simulink model "BEV_Laengsdynamikmodell_v2"  (R2023b)
settings: configuration reference "SharedConfig" (kept outside this file)
undefined symbols (not defined in the file): acc_cycle_flag, Analyse, battery, battery_builder_rtmsupport, config_battery, config_gearbox, config_Inverter, config_motor, config_vehicle, GB, gcbh, gearbox_map, k_FW, ModuleAssembly1, ModuleType1, motormap, motormap2
libraries: powerlib x37, nesl_utility x18, GD_Batterymodel_NSGAII_1_lib x12, BatteryProtection x9, fl_lib x7, dspstat3 x4, simulink x3, eePmsmCurrentReferenceGen x2, spsControlledCurrentSourceLib x2, spsVoltageMeasurementLib x2, batt_lib x1, BatteryBalancing x1
(part 6 of 6)

== matlab function BEV_Laengsdynamikmodell_v2/Variant Subsystem Inverter/Inverter Analytic/Variant Subsystem/IM_Inverter_SiC-MOSFET_Analytic/C2M0025120D ==
  data: io input; udc input; up input; fs input; CPloss_SiC output; CPloss_diode output; costheta input; SPloss_SiC output; SPloss_diode output; T_mosfet input; T_diode input
function [CPloss_SiC,CPloss_diode,SPloss_SiC,SPloss_diode] = SiC_MOSFET(io,udc,up,fs,costheta,T_mosfet,T_diode)
%%%%%%%%%%%%%%%%%%%%%%%%%%% parameter table %%%%%%%%%%%%%%%%%%%%%%%%%%%%%%%
%%%%%%%%%%%%%%%%%%%%%%%%%%% varialbe table %%%%%%%%%%%%%%%%%%%%%%%%%%%%%%%%
%variavle name      meaning,                                                        unit
%io,                operation current                                               (A)
%up,                operation voltage                                               (V)
%udc,               DC bus voltage,                                                 (V)
%fs,                switching frequency,                                            (Hz)
%costheta,          power factor,                                                   (none)
%CPloss_igbt,       conduction loss on IGBT,                                        (W)
%CPloss_diode,      conduction loss on the reverse paralleled diode,                (W)
%SPloss_igbt,       switching loss on IGBT,                                         (W)
%SPloss_diode,      switching loss on the reverse paralleled diode,                 (W)
%%%%%%%%%%%%%%%%%%%%%%%%%%%%%%%%%%%%%%%%%%%%%%%%%%%%%%%%%%%%%%%%%%%%%%%%%%%
parallel = 4;

io = io/parallel;
rdson_max = 0.02;       
alpha = (1.45 - 1)/(150 - 25);
ud_plateau25 = 1;                              % Fig.11; Vth,25 = 2.7
ud_plateau150 = 0.717;                         % Fig.11; Vth,150 = 2.3
%%%%%%%%%%%%%%%%%%%%%%%%%%%% linearization %%%%%%%%%%%%%%%%%%%%%%%%%%%%%%%%
rdson = rdson_max*(1 + alpha/100)^(T_mosfet - 25);
ud_plateau = ud_plateau25 + (ud_plateau25-ud_plateau150)/(25-150)*(T_diode-25);

rd = (-6 - (-3.75))/(-200 - 0) * 1.2;          % engineering calculation use safty margin value, linearization from Fig.10, using Vsd,typ = 3.5;

Eon_SiC = (0.00069/80*(io*(2/pi)))/520*udc;    % linearization from Fig.23; V_DD = 600; Eon(60, 0.0015);
Eoff_SiC = (0.001125/80*(io*(2/pi)))/520*udc;  % linearization from Fig.23; V_DD = 600; Eoff(60, 0.00075);
Eon_diode = 0;
Eoff_diode = 0;
%%%%%%%%%%%%%%%%%%%%%%%%%%%%%%%%%%%%%%%%%%%%%%%%%%%%%%%%%%%%%%%%%%%%%%%%%%%
m = sqrt(2)*up*2/udc;

if io*rdson <= ud_plateau
   CPloss_SiC = rdson*io^2;
   CPloss_diode = 0;
   SPloss_SiC = fs*(Eon_SiC+Eoff_SiC);
   SPloss_diode = fs*(Eon_diode+Eoff_diode);
else
   CPloss_SiC = 2*rdson*io*io*(1/8+m*costheta/3/pi);
   CPloss_diode = sqrt(2)*ud_plateau*io*(1/2/pi-m*costheta/8)+2*rd*io*io*(1/8-m*costheta/3/pi);
   SPloss_SiC = fs*(Eon_SiC+Eoff_SiC);
   SPloss_diode = fs*(Eon_diode+Eoff_diode);
end

CPloss_SiC = CPloss_SiC*parallel;
SPloss_SiC = SPloss_SiC*parallel;
CPloss_diode = CPloss_diode*parallel;
SPloss_diode = SPloss_diode*parallel;

if io == 0
   SPloss_SiC = 0;
   SPloss_diode = 0;
end
end

== matlab function BEV_Laengsdynamikmodell_v2/MATLAB Function1 ==
  data: u input
function fcn(u)
%disp('rpm:')
%disp (u)

== matlab function BEV_Laengsdynamikmodell_v2/Variant Subsystem Gearbox/Gearbox Analytic/Oil Temp/MATLAB Function ==
  data: t input; P_V input; T output
function T = fcn(t, P_V)

coder.extrinsic('evalin');

% Calculate lubricant temperature
ambient_temp = 0;
ambient_temp = evalin('base', 'config_vehicle.ambient_temp');
% 
% if t < (ambient_temp - 273)
%     T = (ambient_temp - 273);
% elseif t <= 70 %Aufwärmphase mit Umgebung < t < 70°C
%     T = abs(P) * 0.0003 + rpm * 0.00004 + t; %Leistungsabhängiger und drehzahlabhängiger Energieeintrag (Temperaturanstieg)
% else %Temperatur t > 70°C -> Wärmeabgabe ~ delta_t und ~ delta_t^2 (mit delta_t = t_gearbox - t_ambient)
%     T = abs(P) * 0.0003 + rpm * 0.00004 + t - (t - ambient_temp + 273) * 0.0002 - (t - ambient_temp + 273)^2 * 0.0000022;
% end

if t < (ambient_temp - 273)
    T = (ambient_temp - 273);
elseif t <= 80 %Aufwärmphase mit Umgebung < t < 70°C
    T =0.000055*P_V + t - (t - ambient_temp + 273) * 0.0003; %Leistungsabhängiger und drehzahlabhängiger Energieeintrag (Temperaturanstieg)
else %Temperatur t > 70°C -> Wärmeabgabe ~ delta_t und ~ delta_t^2 (mit delta_t = t_gearbox - t_ambient)
    T = 0.000088*P_V + t - (t - ambient_temp + 273) * 0.0010 - (t - ambient_temp + 273)^2 * 0.000012;
end

end

== matlab function BEV_Laengsdynamikmodell_v2/Variant Subsystem Inverter/Inverter Analytic/Variant Subsystem/IM_Inverter_SiC-MOSFET_Analytic/MATLAB Function3 ==
  data: u output; T_m input; i output; usq input; usd input; costheta output; n input
function [u, i, costheta] = fcn(T_m, usq, usd, n)

   Lm = 4.5e-4;
   Lr =  0.01571 + Lm;
   p = 3;
   T_e = T_m/p;
   
   if T_m >=0
       id = -sqrt((2*T_e/p*Lr)/(3*p*Lm^2));
   else
       id = sqrt((-2*T_e/p*Lr)/(3*p*Lm^2));
   end
   iq = id;
   i = sqrt(id^2 + iq^2)/2;
   u = sqrt(usq*usq+usd*usd);
   costheta = (usd*id+usq*iq)/u/i;

   if isnan(costheta)
       costheta = 1;
   end

   if n < 0.1
       u = 0;
       i = 0;
       costheta = 1;
   end

end

== matlab function BEV_Laengsdynamikmodell_v2/Current_fix/MATLAB Function3 ==
  data: state input; u input; y output; st output
function [y, st] = fcn(state, u)
z = 0;
st = 0;
u = double(u);

coder.extrinsic('evalin');

z = evalin('base', 'acc_cycle_flag');
if state == 1
    y = state;
else
    if (u == 1) && (z == 1)
        warning("Battery: Voltage went below 0V - Quiting battery simulation for acceleration-cycle")
    elseif (u == 1) && (z ~= 1)
        warning("Battery: Voltage went below 0V - Battery failed in Main Drivingcycle - Stopping simulation")
        st = 1;
    end
    y = u;
end

== matlab function BEV_Laengsdynamikmodell_v2/Variant Subsystem Battery/Battery simplified (R0)/Battery/MATLAB Function3 ==
  settings: updateMethod=DISCRETE
  data: car_current input; parallel_cells input; V0_matCell input; iCell output; numCyclesCell output; socCell output; socParallelAssembly output; temperatureCell output; vCell output; vParallelAssembly output; R0_matCell input; AH_Cell input; thermal_massCell input; AmbientResistance input; InitialSOC input; T_battery input; SOC_vecCell input; T_vecCell input; T_ambient input; time input; P_bat_loss output
function [iCell, numCyclesCell, socCell, socParallelAssembly, temperatureCell, vCell, vParallelAssembly, P_bat_loss] = fcn(car_current, parallel_cells, V0_matCell, R0_matCell, AH_Cell, ...
    thermal_massCell, AmbientResistance, InitialSOC, T_battery, SOC_vecCell, T_vecCell, T_ambient, time)

    % Initialize Parameters
    dt = 1;  % Time step in seconds
    T_target_inital = 298.15;
    alpha = 1.25e-4;
    T_target = T_target_inital + alpha * time;  % Target temperature in K (e.g., 25°C)
    K_p = 0.1;  % Proportional gain for PI controller
    K_i = 0.01;  % Integral gain for PI control
    persistent numCyclesCell_previous soc_previous T_battery_previous integral_error;

    if isempty(soc_previous)
        soc_previous = InitialSOC;  % Set initial state of charge
        numCyclesCell_previous = 0;  % Initial number of cycles
        T_battery_previous = T_battery;  % Initial battery temperature
        integral_error = 0;  % Initialize integral term for PI control
    end

    % Battery Current (car_current as input)
    iCell = car_current / parallel_cells;  % Current flowing through each cell

    % Update State of Charge using Coulomb counting
    if iCell ~= 0
        socCell = soc_previous - (-iCell * dt / (3600 * AH_Cell));  % Updated SOC
    else
        socCell = soc_previous;  % No change if no current
    end
    socCell = max(0, min(socCell, 1));  % Ensure SOC stays within valid range [0, 1]

    % Update cycle count
    delta_soc = soc_previous - socCell;
    numCyclesIncrement = max(0, delta_soc);
    numCyclesCell_previous = numCyclesCell_previous + numCyclesIncrement;
    numCyclesCell = numCyclesCell_previous;
    socParallelAssembly = socCell;

    % Heat Transfer Calculations
    Q_ambient = (T_battery_previous - T_ambient) / AmbientResistance;

    % PI control for dynamic mass flow rate
    error = T_battery_previous - T_target;
    integral_error = integral_error + error * dt;
    mass_dot = max(0, K_p * error + K_i * integral_error);

    % Maximum mass flow rate limit
    Re = 2000; % Laminar flow
    mu = 8.9e-4; % Dynamic viscosity of water
    density = 1000; % Density of water
    D_h = 0.005; % Hydraulic diameter of pipe
    n = 4; % Number of channels
    A = (pi * n * D_h^2) / 4; % Cross-sectional area of channels
    cp = 4184; % Specific heat capacity of water
    v = (Re * mu) / (density * D_h); % Flow velocity of coolant
    
    mass_dot_max = density * A * v;
    mass_dot = min(mass_dot, mass_dot_max);

    Delta_T_initial = 0.03;   % Initial jump in temperature difference
    Delta_T_max = 0.04;       % Maximum temperature difference at steady state
    tau = 10;                 % Time constant, adjust based on system behavior
    beta = 4e-5;
    Temp_difference = Delta_T_initial + (Delta_T_max - Delta_T_initial) * (1 - exp(-time / tau)) + beta*time;

    Q_coolant = mass_dot * cp * Temp_difference;
    Q_total = Q_coolant + Q_ambient;

    % Iterative temperature calculation
    tolerance = 1e-3;
    max_iterations = 100;
    T_battery_new = T_battery_previous;
    iteration = 0;

    while true
        R0_interpolated = interp2(T_vecCell, SOC_vecCell, R0_matCell, T_battery_new, socCell, 'linear');

        % Heat generated
        Q_generated = iCell^2 * (R0_interpolated);
        dT_battery_dt = (Q_generated - Q_total) / thermal_massCell;
        T_battery_new_next = T_battery_previous + dT_battery_dt * dt;

        % Check convergence
        if abs(T_battery_new_next - T_battery_new) < tolerance
            break;
        end
        T_battery_new = T_battery_new_next;
        iteration = iteration + 1;

        if iteration >= max_iterations
            warning('Temperature calculation did not converge within max iterations');
            break;
        end
    end

    T_battery_new = T_battery_new_next;
    temperatureCell = T_battery_new;

    % Interpolated OCV
    V0_interpolated = interp2(T_vecCell, SOC_vecCell, V0_matCell, T_battery_new, socCell, 'linear');

    % Calculate vCell including dynamic effects
    vCell = V0_interpolated - (-iCell * R0_interpolated);

    % Voltage for Parallel Assembly
    vParallelAssembly = vCell;

    % Update previous state variables for the next time step
    soc_previous = socCell;
    T_battery_previous = T_battery_new;
    
    % Ohmic losses
    Q_ohmic = Q_generated;
    % Total losses
    Q_total_loss = Q_ohmic;
    
    P_bat_loss = Q_total_loss;


end

== matlab function BEV_Laengsdynamikmodell_v2/MATLAB Function2 ==
  data: u input
function fcn(u)
%disp('torque')
%disp (u)

== matlab function BEV_Laengsdynamikmodell_v2/Variant Subsystem Inverter/Inverter Simple/MATLAB Function ==
  data: P_inv_loss output; I_dc output; T input; n input; udc input; P_inv_total output; P_mot_total output; P_Terminal input
function [P_inv_loss, I_dc, P_inv_total, P_mot_total]= fcn(T, n, udc, P_Terminal)

    correction_faktor = 1;

    P_inv_total = P_Terminal;
    I_dc = P_inv_total/udc;
    P_mot_total = (2*T*pi*n/60+P_inv_total)/2;
    P_inv_loss = correction_faktor * (P_inv_total - P_mot_total);

end

== matlab function BEV_Laengsdynamikmodell_v2/Variant Subsystem Gearbox/Gearbox Lookup-Table/Oil Temp Gao/MATLAB Function ==
  data: t input; P input; T output; rpm input
function T = fcn(t, P, rpm)

coder.extrinsic('evalin');

% Calculate lubricant temperature
ambient_temp = 0;
ambient_temp = evalin('base', 'config_vehicle.ambient_temp');

% if t < (ambient_temp - 273)
%     T = (ambient_temp - 273);
% elseif t <= 75
%     T = abs(P) * 0.005 + t - (t - ambient_temp + 273)* 0.001;
% else
%     T = abs(P) * 0.005 + t - (t - 75) * 0.002 - (t - ambient_temp + 273)* 0.001;
% end

if t < (ambient_temp - 273)
    T = (ambient_temp - 273);
elseif t <= 70 %Aufwärmphase mit Umgebung < t < 70°C
    T = abs(P) * 0.0003 + rpm * 0.00004 + t; %Leistungsabhängiger und drehzahlabhängiger Energieeintrag (Temperaturanstieg)
else %Temperatur t > 70°C -> Wärmeabgabe ~ delta_t und ~ delta_t^2 (mit delta_t = t_gearbox - t_ambient)
    T = abs(P) * 0.0003 + rpm * 0.00004 + t - (t - ambient_temp + 273) * 0.0002 - (t - ambient_temp + 273)^2 * 0.0000022;
end

end

== matlab function BEV_Laengsdynamikmodell_v2/Variant Subsystem Gearbox/Gearbox Analytic/Variant Subsystem Analytic GB/Zweistufig_Koaxial/MATLAB Function ==
  data: P_V output double size=1; Mrad input; nrad input; Temp input; GB parameter
function P_V = Getriebe_Einstufig_Achsparallel(Mrad, nrad, Temp, GB)

if nrad == 0
    P_V = 0;
else
    P_V = Getrieberechnung_koaxial(GB,Mrad,nrad,Temp);
end

end

== matlab function BEV_Laengsdynamikmodell_v2/Variant Subsystem Motor/Motor Lookup-Table/MATLAB Function2 ==
  data: u input; y output
function y = fcn(u)

if isnan(u)
    warning('P_motor_111 is NaN. Setting it to 0.');
    y = 0;
else
    y = u;
end

== matlab function BEV_Laengsdynamikmodell_v2/Variant Subsystem Motor/Motor Lookup-Table/MATLAB Function1 ==
  data: u input; y output
function y = fcn(u)

if isnan(u)
    warning('P_bmotor_2 is NaN. Setting it to 0.');
    y = 0;
else
    y = u;
end

== matlab function BEV_Laengsdynamikmodell_v2/Variant Subsystem Inverter/Inverter Analytic/Variant Subsystem/IM_Inverter_IGBT_Analytic/MATLAB Function ==
  data: t input; udc input; w_mech input; u_sq output; u_sd output
function [u_sq, u_sd] = fcn(t, udc, w_mech)
    
    p = 3; %pole pairs
    
    V_line = udc/2;
    V_phase = V_line/sqrt(3);
    w_elect = p * w_mech;
    
    V_a = V_phase * sin(w_elect * t);
    V_b = V_phase * sin(w_elect * t - 2*pi/3);
    V_c = V_phase * sin(w_elect * t + 2*pi/3);

    % Transformation from abc to dq reference frame
    % Assuming stator flux-oriented control with d-axis aligned with rotor flux
    theta_e = w_elect * t; % Electrical angle
    
    % Clarke transformation to alpha-beta reference frame
    V_alpha = (2/3) * (V_a - 0.5 * (V_b + V_c));
    V_beta = (2/3) * ((sqrt(3)/2) * (V_b - V_c));
    
    % Park transformation to d-q reference frame
    u_sd = V_alpha * cos(theta_e) + V_beta * sin(theta_e);
    u_sq = -V_alpha * sin(theta_e) + V_beta * cos(theta_e);

end

== matlab function BEV_Laengsdynamikmodell_v2/Variant Subsystem Gearbox/Gearbox Analytic/Oil Temp Gao/MATLAB Function ==
  data: t input; P input; T output; rpm input
function T = fcn(t, P, rpm)

coder.extrinsic('evalin');

% Calculate lubricant temperature
ambient_temp = 0;
ambient_temp = evalin('base', 'config_vehicle.ambient_temp');

% if t < (ambient_temp - 273)
%     T = (ambient_temp - 273);
% elseif t <= 75
%     T = abs(P) * 0.005 + t - (t - ambient_temp + 273)* 0.001;
% else
%     T = abs(P) * 0.005 + t - (t - 75) * 0.002 - (t - ambient_temp + 273)* 0.001;
% end

if t < (ambient_temp - 273)
    T = (ambient_temp - 273);
elseif t <= 70 %Aufwärmphase mit Umgebung < t < 70°C
    T = abs(P) * 0.0003 + rpm * 0.00004 + t; %Leistungsabhängiger und drehzahlabhängiger Energieeintrag (Temperaturanstieg)
else %Temperatur t > 70°C -> Wärmeabgabe ~ delta_t und ~ delta_t^2 (mit delta_t = t_gearbox - t_ambient)
    T = abs(P) * 0.0003 + rpm * 0.00004 + t - (t - ambient_temp + 273) * 0.0002 - (t - ambient_temp + 273)^2 * 0.0000022;
end

end

== matlab function BEV_Laengsdynamikmodell_v2/Variant Subsystem Gearbox/Gearbox Analytic/Variant Subsystem Analytic GB/Zweistufig_Achsparallel/MATLAB Function ==
  data: P_V output double size=1; Mrad input; nrad input; Temp input; GB parameter
function P_V  = Getriebe_Zweistufig_Achsparallel(Mrad, nrad, Temp, GB)

if nrad == 0
    P_V = 0;
else
    [P_V] = Getrieberechnung(GB,Mrad,nrad,Temp);
end

end

== matlab function BEV_Laengsdynamikmodell_v2/Variant Subsystem Motor/Motor Lookup-TableOneMotor/MATLAB Function2 ==
  data: u input; y output
function y = fcn(u)

if isnan(u)
    warning('P_motor_111 is NaN. Setting it to 0.');
    y = 0;
else
    y = u;
end

== matlab function BEV_Laengsdynamikmodell_v2/MATLAB Function3 ==
  data: u input; y output
function y = fcn(u)

if isnan(u)
    warning('P_inverter is NaN. Setting it to 0.');
    y = 0;
else
    y = u;
end

== matlab function BEV_Laengsdynamikmodell_v2/Variant Subsystem Battery/Battery Global Drive/Battery/MATLAB Function ==
  data: u input; y output
function y = fcn(u)
if u == 1
    warning("Battery: SOC went below allowed value")
end
y = u;

== matlab function BEV_Laengsdynamikmodell_v2/Variant Subsystem Battery/Battery Global Drive/Battery/MATLAB Function1 ==
  data: u input; y output
function y = fcn(u)
if u == 1
    warning("Battery: LE drew more current then allowed")
end
y = u;

== matlab function BEV_Laengsdynamikmodell_v2/Variant Subsystem Battery/Battery Global Drive/Battery/battery voltage checker - 50%/MATLAB Function2 ==
  data: u input; y output; d input; st output; z input
function [y,st]= fcn(u, d, z)

y = u;
st = 0;

if u == 1 && d == 0
    if z == 1
    warning("Battery: Voltage went below 50%")
    else
        warning("Battery: Stopping simulation as voltage went below 50% in Main Driving Cycle")
        st = 1;
    end
end

== matlab function BEV_Laengsdynamikmodell_v2/Variant Subsystem Battery/Battery simplified (R0)/Battery/MATLAB Function ==
  data: u input; y output
function y = fcn(u)
if u == 1
    warning("Battery: SOC went below allowed value")
end
y = u;

== matlab function BEV_Laengsdynamikmodell_v2/Variant Subsystem Battery/Battery simplified (R0)/Battery/MATLAB Function1 ==
  data: u input; y output
function y = fcn(u)
if u == 1
    warning("Battery: LE drew more current then allowed")
end
y = u;

== matlab function BEV_Laengsdynamikmodell_v2/Variant Subsystem Battery/Battery simplified (R0)/Battery/battery voltage checker - 50%/MATLAB Function2 ==
  data: u input; y output; d input; st output; z input
function [y,st]= fcn(u, d, z)

y = u;
st = 0;

if u == 1 && d == 0
    if z == 1
    warning("Battery: Voltage went below 50%")
    else
        warning("Battery: Stopping simulation as voltage went below 50% in Main Driving Cycle")
        st = 1;
    end
end

== matlab function BEV_Laengsdynamikmodell_v2/Variant Subsystem Inverter/Inverter Analytic/Variant Subsystem/PMSM_Inverter_IBGT_Analytic/Analytic1 ==
  data: id_ref input; u output; i output; iq_ref input; costheta output; n input
function [u, i, costheta] =  u(id_ref,iq_ref, n)

    % Updated Motor Parameters based on provided values
    p = 6; % Number of pole pairs (from the provided data)
    psi_pm = 0.0347; % Permanent magnet flux linkage in Wb
    Ld = 0.0000436; % d-axis inductance in H
    Lq = 0.0000975; % q-axis inductance in H
    Rs = 0.0049; % Stator resistance in Ohms
    we = n*p/60*2*pi;

    is_ref = sqrt(id_ref^2 + iq_ref^2);

    isd = 1/(4*(Lq - Ld)) * (psi_pm - sqrt(psi_pm^2 + 8*is_ref^2*(Lq - Ld)^2));
    isq = sqrt(is_ref^2 - isd^2);

    usd = Rs*isd - we*Lq*isq;
    usq = Rs*isq + we*Ld*isd + we*psi_pm;
    % if u > urate*sqrt(2)
    %     if abs(n*T*2*pi/60) >= Prate
    %         Tout = Prate/(n/60*2*pi);
    %     else
    %         Tout = T;
    %     end
    %     isd = id_ref;
    %     isq = iq_ref;
    %     usd = ud_ref;
    %     usq = uq_ref;
    % end

    i = sqrt(isq*isq+isd*isd);
    u = sqrt(usq*usq+usd*usd);
    costheta = (usd*isd+usq*isq)/u/i;

    if isnan(costheta)
        costheta = 1;
    end
    if n < 0.1
        u = 0;
        i = 0;
        % Tout = 0;
        costheta = 1;
    end
    % if Tout ~= T
    %     Tout = T;
    % end
end

== matlab function BEV_Laengsdynamikmodell_v2/Variant Subsystem Inverter/Inverter Analytic/Variant Subsystem/PMSM_Inverter_SiC-MOSFET_Analytic/C2M0025120D ==
  data: io input; udc input; up input; fs input; CPloss_SiC output; CPloss_diode output; costheta input; SPloss_SiC output; SPloss_diode output; T_mosfet input; T_diode input
function [CPloss_SiC,CPloss_diode,SPloss_SiC,SPloss_diode] = SiC_MOSFET(io,udc,up,fs,costheta,T_mosfet,T_diode)
%%%%%%%%%%%%%%%%%%%%%%%%%%% parameter table %%%%%%%%%%%%%%%%%%%%%%%%%%%%%%%
%%%%%%%%%%%%%%%%%%%%%%%%%%% varialbe table %%%%%%%%%%%%%%%%%%%%%%%%%%%%%%%%
%variavle name      meaning,                                                        unit
%io,                operation current                                               (A)
%up,                operation voltage                                               (V)
%udc,               DC bus voltage,                                                 (V)
%fs,                switching frequency,                                            (Hz)
%costheta,          power factor,                                                   (none)
%CPloss_igbt,       conduction loss on IGBT,                                        (W)
%CPloss_diode,      conduction loss on the reverse paralleled diode,                (W)
%SPloss_igbt,       switching loss on IGBT,                                         (W)
%SPloss_diode,      switching loss on the reverse paralleled diode,                 (W)
%%%%%%%%%%%%%%%%%%%%%%%%%%%%%%%%%%%%%%%%%%%%%%%%%%%%%%%%%%%%%%%%%%%%%%%%%%%
parallel = 4;

io = io/parallel;
rdson_max = 0.02;       
alpha = (1.45 - 1)/(150 - 25);
ud_plateau25 = 1;                              % Fig.11; Vth,25 = 2.7
ud_plateau150 = 0.717;                         % Fig.11; Vth,150 = 2.3
%%%%%%%%%%%%%%%%%%%%%%%%%%%% linearization %%%%%%%%%%%%%%%%%%%%%%%%%%%%%%%%
rdson = rdson_max*(1 + alpha/100)^(T_mosfet - 25);
ud_plateau = ud_plateau25 + (ud_plateau25-ud_plateau150)/(25-150)*(T_diode-25);

rd = (-6 - (-3.75))/(-200 - 0) * 1.2;          % engineering calculation use safty margin value, linearization from Fig.10, using Vsd,typ = 3.5;

Eon_SiC = (0.00069/80*(io*(2/pi)))/520*udc;    % linearization from Fig.23; V_DD = 600; Eon(60, 0.0015);
Eoff_SiC = (0.001125/80*(io*(2/pi)))/520*udc;  % linearization from Fig.23; V_DD = 600; Eoff(60, 0.00075);
Eon_diode = 0;
Eoff_diode = 0;
%%%%%%%%%%%%%%%%%%%%%%%%%%%%%%%%%%%%%%%%%%%%%%%%%%%%%%%%%%%%%%%%%%%%%%%%%%%
m = sqrt(2)*up*2/udc;

if io*rdson <= ud_plateau
   CPloss_SiC = rdson*io^2;
   CPloss_diode = 0;
   SPloss_SiC = fs*(Eon_SiC+Eoff_SiC);
   SPloss_diode = fs*(Eon_diode+Eoff_diode);
else
   CPloss_SiC = 2*rdson*io*io*(1/8+m*costheta/3/pi);
   CPloss_diode = sqrt(2)*ud_plateau*io*(1/2/pi-m*costheta/8)+2*rd*io*io*(1/8-m*costheta/3/pi);
   SPloss_SiC = fs*(Eon_SiC+Eoff_SiC);
   SPloss_diode = fs*(Eon_diode+Eoff_diode);
end

CPloss_SiC = CPloss_SiC*parallel;
SPloss_SiC = SPloss_SiC*parallel;
CPloss_diode = CPloss_diode*parallel;
SPloss_diode = SPloss_diode*parallel;

if io == 0
   SPloss_SiC = 0;
   SPloss_diode = 0;
end
end

== matlab function BEV_Laengsdynamikmodell_v2/Variant Subsystem Inverter/Inverter Analytic/Variant Subsystem/PMSM_Inverter_IBGT_Analytic/Change parameters from datasheet here1 ==
  data: ic input; udc input; up input; fs input; CPloss_igbt output; CPloss_diode output; costheta input; Eon_igbt_nom input; Eoff_igbt_nom input; Erec_diode_nom input; SPloss_igbt output; SPloss_diode output; T_igbt input; T_diode input
function [CPloss_igbt,CPloss_diode,SPloss_igbt,SPloss_diode] = IGBT(ic,udc,up,fs,costheta,Eon_igbt_nom, Eoff_igbt_nom, Erec_diode_nom, T_igbt, T_diode)
%%%%%%%%%%%%%%%%%%%%%%%%%%% parameter table %%%%%%%%%%%%%%%%%%%%%%%%%%%%%%%
%%%%%%%%%%%%%%%%%%%%%%%%%%% varialbe table %%%%%%%%%%%%%%%%%%%%%%%%%%%%%%%%
% variavle name      meaning,                                                        unit
% ic,                operation current peak                                          (A)
% up,                operation voltage peak                                          (V)
% udc,               DC bus voltage,                                                 (V)
% fs,                switching frequency,                                            (Hz)
% costheta,          power factor,                                                   (none)
% CPloss_igbt,       conduction loss on IGBT,                                        (W)
% CPloss_diode,      conduction loss on the reverse paralleled diode,                (W)
% SPloss_igbt,       switching loss on IGBT,                                         (W)
% SPloss_diode,      switching loss on the reverse paralleled diode,                 (W)
%%%%%%%%%%%%%%%%%%%%%%%%%%%%%%%%%%%%%%%%%%%%%%%%%%%%%%%%%%%%%%%%%%%%%%%%%%%
parallel = 1;

ic = ic/parallel;

icn = 450;
uce_test = 400;
ifn = 450;
uf_test = 400;

T25 = 25;
T175 = 175;
uce0 = 0.75;
rc25 = 0.0005;
rc175 = 0.00089;
kCE = (rc175-rc25)/(T175-T25);
ud0 = 0.95;
rd25 = 0.00067;
rd175 = 0.00075;
kD = (rd175-rd25)/(T175-T25);
%%
rc = rc25 + (T_igbt - 25)*kCE;  
rd = rd25 + (T_diode - 25)*kD; 
uce = uce0 + ic*rc;             
uf = ud0 + ic*rd;            

m = up*sqrt(2)*2/udc; 

Eon_igbt = Eon_igbt_nom * ic/icn * udc/uce_test;    
Eoff_igbt = Eoff_igbt_nom * ic/ifn * udc/uce_test;         
Erec_diode = Erec_diode_nom * ic/ifn * udc/uf_test; 

CPloss_igbt = sqrt(2)*uce*ic*(1/2/pi+m*costheta/8) + 2*rc*ic*ic*(1/8+m*costheta/3/pi);
CPloss_diode = sqrt(2)*uf*ic*(1/2/pi-m*costheta/8) + 2*rd*ic*ic*(1/8-m*costheta/3/pi);
SPloss_igbt = fs*(Eon_igbt+Eoff_igbt);
SPloss_diode = fs*Erec_diode;

CPloss_igbt = CPloss_igbt*parallel;
CPloss_diode = CPloss_diode*parallel;
SPloss_igbt = SPloss_igbt*parallel;
SPloss_diode = SPloss_diode*parallel;

if ic == 0
    SPloss_igbt = 0;
    SPloss_diode = 0;
end
end

== matlab function BEV_Laengsdynamikmodell_v2/Variant Subsystem Inverter/Inverter Analytic/Variant Subsystem/PMSM_Inverter_SiC-MOSFET_Analytic/Analytic1 ==
  data: id_ref input; u output; i output; iq_ref input; costheta output; n input
function [u, i, costheta] =  u(id_ref,iq_ref, n)

    % Updated Motor Parameters based on provided values
    p = 6; % Number of pole pairs (from the provided data)
    psi_pm = 0.0347; % Permanent magnet flux linkage in Wb
    Ld = 0.0000436; % d-axis inductance in H
    Lq = 0.0000975; % q-axis inductance in H
    Rs = 0.0049; % Stator resistance in Ohms
    we = n*p/60*2*pi;
    urate = 142.56;

    is_ref = sqrt(id_ref^2 + iq_ref^2);

    isd = 1/(4*(Lq - Ld)) * (psi_pm - sqrt(psi_pm^2 + 8*is_ref^2*(Lq - Ld)^2));
    isq = sqrt(is_ref^2 - isd^2);

    usd = Rs*isd - we*Lq*isq;
    usq = Rs*isq + we*Ld*isd + we*psi_pm;

    i = sqrt(isq*isq+isd*isd);
    u = sqrt(usq*usq+usd*usd);
    
    if u > urate*sqrt(2)
        % if abs(n*T*2*pi/60) >= Prate
        %     Tout = Prate/(n/60*2*pi);
        % else
        %     Tout = T;
        % end
        isd = id_ref;
        isq = iq_ref;
        % usd = ud_ref;
        % usq = uq_ref;
    end

    i = sqrt(isq*isq+isd*isd);
    u = sqrt(usq*usq+usd*usd);
    costheta = (usd*isd+usq*isq)/u/i;

    if isnan(costheta)
        costheta = 1;
    end
    if n < 0.1
        u = 0;
        i = 0;
        % Tout = 0;
        costheta = 1;
    end
    % if Tout ~= T
    %     Tout = T;
    % end
end

== matlab function BEV_Laengsdynamikmodell_v2/Variant Subsystem Gearbox/Gearbox Analytic/Variant Subsystem Analytic GB/Einstufig_Achsparallel/MATLAB Function ==
  data: P_V output double size=1; Mrad input; nrad input; Temp input; GB parameter
function P_V = Getriebe_Einstufig_Achsparallel(Mrad, nrad, Temp, GB)

if nrad == 0
    P_V = 0;
else
    P_V = Getrieberechnung_Einstufig(GB,Mrad,nrad, Temp);
end

end

== matlab function BEV_Laengsdynamikmodell_v2/Variant Subsystem Battery/Battery Analytic (RC3)/Battery/MATLAB Function ==
  data: u input; y output
function y = fcn(u)
if u == 1
    warning("Battery: SOC went below allowed value")
end
y = u;
